simulink model "lab2"  (R2018a)
settings: Solver=ode23tb  StartTime=0.0  StopTime=5.0  MaxStep=5e-005  RelTol=1e-3
libraries: powerlib x16, simulink x1, powerlib_extras x1
settings Model: Creator=KJ_Fa  LastModifiedBy=KJ_Fa
settings CodeAppCC: StateflowObjectComments=on

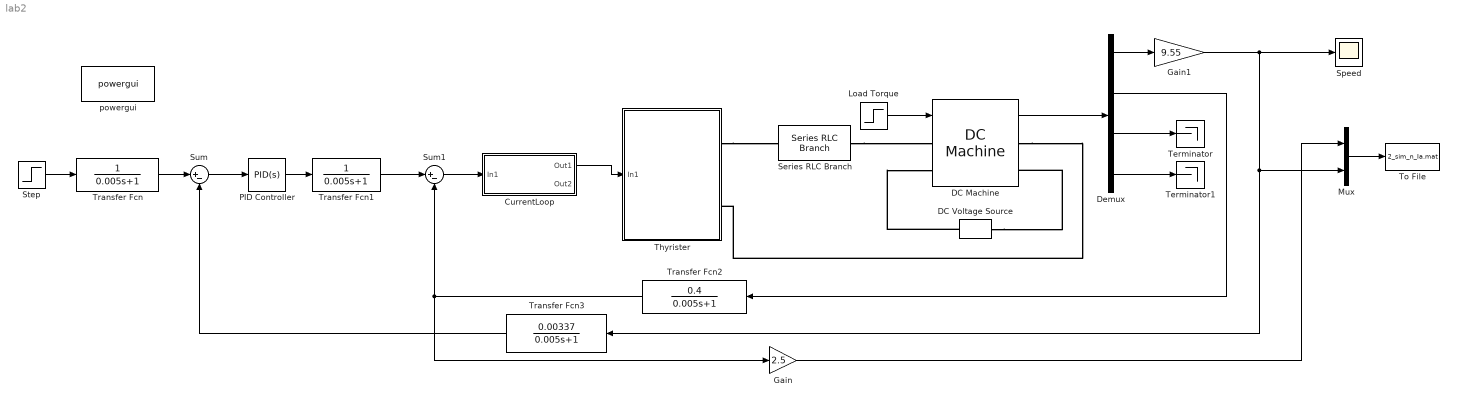
== system lab2 ==
  "CurrentLoop " : Subsystem
  DC Machine : powerlib/Machines/DC Machine  PresetModel=No  MechanicalLoad=Torque TL  FieldType=Wound  ShowDetailedParameters=on  MeasurementBus=off  RLa="[1.92  0.01]"  RLf="[ 200  120]"  Laf=1.25  MachineConstant=Torque constant (N.m/A)  Ke=1.8  Kt=1.8  J=0.204  Bm=0.01  Tf=2  w0=0.1  Ifinit=1  TsPowergui=0  TsBlock=-1
  DC Voltage Source : powerlib/Electrical Sources/DC Voltage Source  Amplitude=200  Measurements=None
  Demux : Demux
  Gain : Gain  Gain=2.5
  Gain1 : Gain  Gain=9.55
  Load Torque : Step  Time=3  Before=10  After=18  SampleTime=0
  Mux : Mux  Inputs=2
  PID Controller : simulink/Continuous/PID Controller  Controller=PID  TimeDomain=Continuous-time  SampleTime=-1  IntegratorMethod=Forward Euler  FilterMethod=Forward Euler  Form=Parallel  UseFilter=on  ControllerParametersSource=internal  P=66.24  I=722.31  D=0  N=100  InitialConditionSource=internal  InitialConditionForIntegrator=0  InitialConditionForFilter=0  ExternalReset=none  LimitOutput=on  UpperSaturationLimit=8  LowerSaturationLimit=-8  LinearizeAsGain=on  AntiWindupMode=clamping  Kb=1  TrackingMode=off  Kt=1  PParamMin=[]  PParamMax=[]  IParamMin=[]  IParamMax=[]  DParamMin=[]  DParamMax=[]  NParamMin=[]  NParamMax=[]  KbParamMin=[]  KbParamMax=[]  KtParamMin=[]  KtParamMax=[]  POutMin=[]  POutMax=[]  IOutMin=[]  IOutMax=[]  DOutMin=[]  DOutMax=[]  NOutMin=[]  NOutMax=[]  KbOutMin=[]  KbOutMax=[]  KtOutMin=[]  KtOutMax=[]  IntegratorOutMin=[]  IntegratorOutMax=[]  FilterOutMin=[]  FilterOutMax=[]  SumOutMin=[]  SumOutMax=[]  SumI1OutMin=[]  SumI1OutMax=[]  SumI2OutMin=[]  SumI2OutMax=[]  SumI3OutMin=[]  SumI3OutMax=[]  SumDOutMin=[]  SumDOutMax=[]  SaturationOutMin=[]  SaturationOutMax=[]  IntegratorContinuousStateAttributes=''  IntegratorStateMustResolveToSignalObject=off  IntegratorRTWStateStorageClass=Auto  FilterContinuousStateAttributes=''  FilterStateMustResolveToSignalObject=off  FilterRTWStateStorageClass=Auto  DifferentiatorICPrevScaledInput=0  DifferentiatorOutMin=[]  DifferentiatorOutMax=[]  FilterDiffOutCoefMin=[]  FilterDiffOutCoefMax=[]  SumDenOutMin=[]  SumDenOutMax=[]  SumNumOutMin=[]  SumNumOutMax=[]  ReciprocalOutMin=[]  ReciprocalOutMax=[]  DivideOutMin=[]  DivideOutMax=[]  TunerSelectOption=Transfer Function Based (PID Tuner App)
  Series RLC Branch : powerlib/Elements/Series RLC Branch  LConnTagsString=__new0  RConnTagsString=__new0  BranchType=L  Resistance=1  Inductance=0.1  SetiL0=off  InitialCurrent=0  Capacitance=1e-6  Setx0=off  InitialVoltage=0  Measurements=None
  Speed : Scope
  Step : Step  Time=0  After=5  SampleTime=0
  Sum : Sum  Inputs=|+-
  Sum1 : Sum  Inputs=|+-
  Terminator : Terminator
  Terminator1 : Terminator
  Thyrister : Subsystem
  To File : ToFile  Filename=2_sim_n_Ia.mat  MatrixName=signals
  Transfer Fcn : TransferFcn  Denominator=[0.005 1]
  Transfer Fcn1 : TransferFcn  Denominator=[0.005 1]
  Transfer Fcn2 : TransferFcn  Numerator=[0.4]  Denominator=[0.005 1]
  Transfer Fcn3 : TransferFcn  Numerator=[0.00337]  Denominator=[0.005 1]
  powergui : powerlib/powergui  Priority=1  SimulationMode=Discrete  SampleTime=5e-005  frequency=60  Iterations=50  frequencyindice=50  Pbase=100e6  ErrMax=1e-4  UnitsV=kV  UnitsW=MW  buscounter=0  FunctionMessages=off  echomessages=off  EnableUseOfTLC=off  CurrentSourceSwitches=off  DisableSnubberDevices=off  DisableRonSwitches=off  DisableVfSwitches=off  DisplayEquations=off  SolverType=Tustin/Backward Euler (TBE)  Interpol=off  ExternalGateDelay=off  methode=off  Ts=100  x0status=blocks  SPID=on  SwTol=0  HookPort=off  RestoreLinks=warning  ResistiveCurrentMeasurement=off  Frange=[0:2:500]  Ylog=off  Xlog=on  ShowGrid=off  save=off  variable=ZData  structure=0  ZoomFFT=off  StartTime=0.0  cycles=1  DisplayStyle=1  fundamental=60  FreqAxis=off  MaxFrequency=1000  frequencyindicesteady=1  RmsSteady=1  display=off
  wires:
  Step/1 -> Transfer Fcn/1
  Transfer Fcn/1 -> Sum/1
  Sum/1 -> PID Controller/1
  PID Controller/1 -> Transfer Fcn1/1
  Transfer Fcn1/1 -> Sum1/1
  Sum1/1 -> "CurrentLoop "/1(In1)
  "CurrentLoop "/1(Out1) -> Thyrister/1(In1)
  Load Torque/1 -> DC Machine/1
  DC Machine/1 -> Demux/1
  Demux/3 -> Terminator/1
  Demux/4 -> Terminator1/1
  Transfer Fcn2/1 -> Gain/1, Sum1/2
  Transfer Fcn3/1 -> Sum/2
  Demux/2 -> Transfer Fcn2/1
  Demux/1 -> Gain1/1
  Gain1/1 -> Transfer Fcn3/1, Mux/2, Speed/1
  Mux/1 -> To File/1
  Gain/1 -> Mux/1
  connections:
  Thyrister/RConn1 -- Series RLC Branch/LConn1
  Series RLC Branch/RConn1 -- DC Machine/LConn1
  DC Machine/RConn1 -- Thyrister/RConn2
  DC Voltage Source/RConn1 -- DC Machine/LConn2
  DC Voltage Source/LConn1 -- DC Machine/RConn2

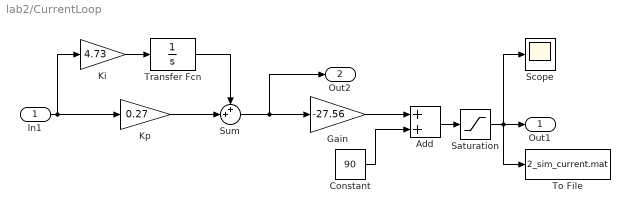
== system lab2/CurrentLoop  ==
  In1 : Inport
  Add : Sum
  Constant : Constant  Value=90
  Gain : Gain  Gain=-27.56
  Ki : Gain  Gain=4.73
  Kp : Gain  Gain=0.27
  Saturation : Saturate  UpperLimit=90  LowerLimit=0
  Scope : Scope
  Sum : Sum  Inputs=++|
  To File : ToFile  Filename=2_sim_current.mat  MatrixName=signals
  Transfer Fcn : TransferFcn  Denominator=[1 0]
  Out1 : Outport
  Out2 : Outport  Port=2
  wires:
  Constant/1 -> Add/2
  Ki/1 -> Transfer Fcn/1
  In1/1 -> Ki/1, Kp/1
  Sum/1 -> Gain/1, Out2/1
  Gain/1 -> Add/1
  Add/1 -> Saturation/1
  Kp/1 -> Sum/2
  Transfer Fcn/1 -> Sum/1
  Saturation/1 -> Out1/1, Scope/1, To File/1

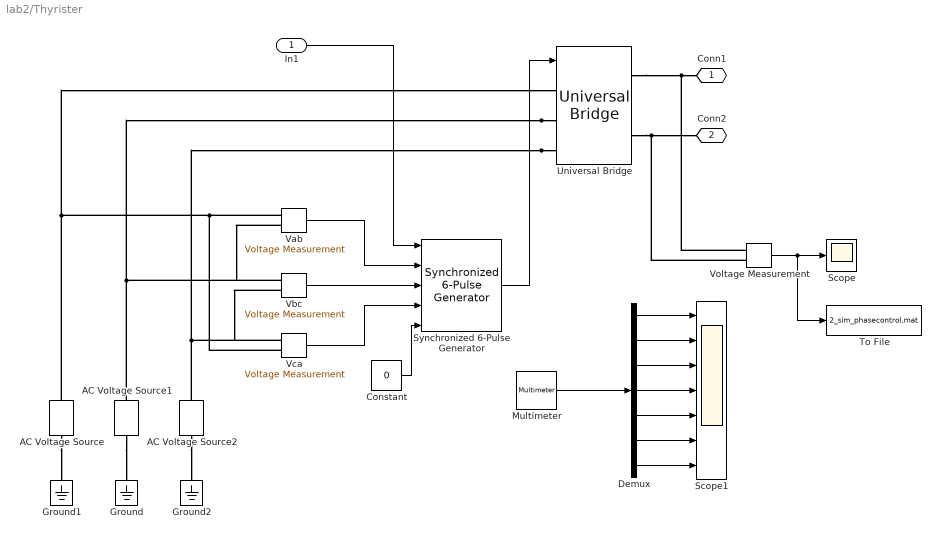
== system lab2/Thyrister ==
  In1 : Inport
  AC Voltage Source : powerlib/Electrical Sources/AC Voltage Source  Amplitude=150  Phase=0  Frequency=50  SampleTime=0  Measurements=None  BusType=swing  Pref=10e3  Qref=0  Qmin=-inf  Qmax=+inf
  AC Voltage Source1 : powerlib/Electrical Sources/AC Voltage Source  Amplitude=150  Phase=-120  Frequency=50  SampleTime=0  Measurements=None  BusType=swing  Pref=10e3  Qref=0  Qmin=-inf  Qmax=+inf
  AC Voltage Source2 : powerlib/Electrical Sources/AC Voltage Source  Amplitude=150  Phase=120  Frequency=50  SampleTime=0  Measurements=None  BusType=swing  Pref=10e3  Qref=0  Qmin=-inf  Qmax=+inf
  Constant : Constant  Value=0
  Demux : Demux  Outputs=7
  Ground : powerlib/Elements/Ground  LConnTagsString=a
  Ground1 : powerlib/Elements/Ground  LConnTagsString=a
  Ground2 : powerlib/Elements/Ground  LConnTagsString=a
  Multimeter : powerlib/Measurements/Multimeter  PhasorSimulation=off  OutputType=Complex  sel=[1 2 3 4 5 6 10]  L=16  Gain=[1 1 1 1 1 1 1]  yselected={'Usw1: Thyrister/Universal Bridge','Usw2: Thyrister/Universal Bridge','Usw3: Thyrister/Universal Bridge','Usw4: Thyrister/Universal Bridge','Usw5: Thyrister/Universal Bridge','Usw6: Thyrister/Universal Bridge','Udc: Thyrister/Universal Bridge'};  PSBOutputType=1  PSBequivalent=0  AxesSetting=[0,0.1,-100,100]  Display=0  SavedBlockNames=-11
  Scope : Scope
  Scope1 : Scope  NumInputPorts=7
  Synchronized 6-Pulse Generator : powerlib_extras/Control  Blocks/Synchronized 6-Pulse Generator  freq=50  pwidth=20  Double_Pulse=on
  To File : ToFile  Filename=2_sim_phasecontrol.mat  MatrixName=signals
  Universal Bridge : powerlib/Power Electronics/Universal Bridge  Arms=3  SnubberResistance=1e5  SnubberCapacitance=inf  Device=Thyristors  Ron=1e-3  Lon=0  ForwardVoltages="[  0  0  ]"  ForwardVoltage=0  GTOparameters=[ 10e-6 , 20e-6 ]  IGBTparameters=[ 1e-6 , 2e-6 ]  Measurements=All voltages and currents  Measurements_2=None  converterType=Rectifier
  Vab : powerlib/Measurements/Voltage Measurement  PhasorSimulation=off  OutputType=Complex  PSBequivalent=0
  Vbc : powerlib/Measurements/Voltage Measurement  PhasorSimulation=off  OutputType=Complex  PSBequivalent=0
  Vca : powerlib/Measurements/Voltage Measurement  PhasorSimulation=off  OutputType=Complex  PSBequivalent=0
  Voltage Measurement : powerlib/Measurements/Voltage Measurement  PhasorSimulation=off  OutputType=Complex  PSBequivalent=0
  Conn1 : PMIOPort  Side=Right
  Conn2 : PMIOPort  Port=2  Side=Right
  wires:
  Synchronized 6-Pulse Generator/1 -> Universal Bridge/1
  Constant/1 -> Synchronized 6-Pulse Generator/5
  Vab/1 -> Synchronized 6-Pulse Generator/2
  Vbc/1 -> Synchronized 6-Pulse Generator/3
  Vca/1 -> Synchronized 6-Pulse Generator/4
  In1/1 -> Synchronized 6-Pulse Generator/1
  Voltage Measurement/1 -> Scope/1, To File/1
  Multimeter/1 -> Demux/1
  Demux/1 -> Scope1/1
  Demux/2 -> Scope1/2
  Demux/3 -> Scope1/3
  Demux/4 -> Scope1/4
  Demux/5 -> Scope1/5
  Demux/6 -> Scope1/6
  Demux/7 -> Scope1/7
  connections:
  Vab/LConn1 -- Vca/LConn2 -- AC Voltage Source/RConn1 -- Universal Bridge/LConn1
  Universal Bridge/LConn2 -- AC Voltage Source1/RConn1 -- Vab/LConn2 -- Vbc/LConn1
  Universal Bridge/LConn3 -- AC Voltage Source2/RConn1 -- Vbc/LConn2 -- Vca/LConn1
  Universal Bridge/RConn1 -- Voltage Measurement/LConn1 -- Conn1/RConn1
  Universal Bridge/RConn2 -- Voltage Measurement/LConn2 -- Conn2/RConn1
  AC Voltage Source1/LConn1 -- Ground/LConn1
  AC Voltage Source/LConn1 -- Ground1/LConn1
  AC Voltage Source2/LConn1 -- Ground2/LConn1
